simulink model "mpc_control_sim"  (R2019b)
settings: Solver=FixedStepAuto  StartTime=0.0  StopTime=72  FixedStep=h  RelTol=1e-3
values from neighbouring files (symbols this model uses):
  h = 0.1    [Example_9_Tracking_Delta_Input_Formulation.m]    (also in dyn_dist_mpc_control.m = 0.01; dyn_mpc_control.m = 0.01; dyn_pid_control.m = 0.01; init.m = 0.05)
  robot_sys_ss = lateral_2_dof_model_continuous_time(h, robot_vel, 0)    [Example_9_Tracking_Delta_Input_Formulation.m]    (also in dyn_dist_mpc_control.m = c2d(robot_sys_ss, h); dyn_mpc_control.m = c2d(robot_sys_ss, h); mpc_control.m = c2d(robot_sys_ss, h); pid_control.m = c2d(robot_sys_ss, h))
libraries: mpclib x1
settings Model: Creator=faaizz  LastModifiedBy=faaizz
settings SFSimCC: CustomCodeUndefinedFunction=UseInterfaceOnly

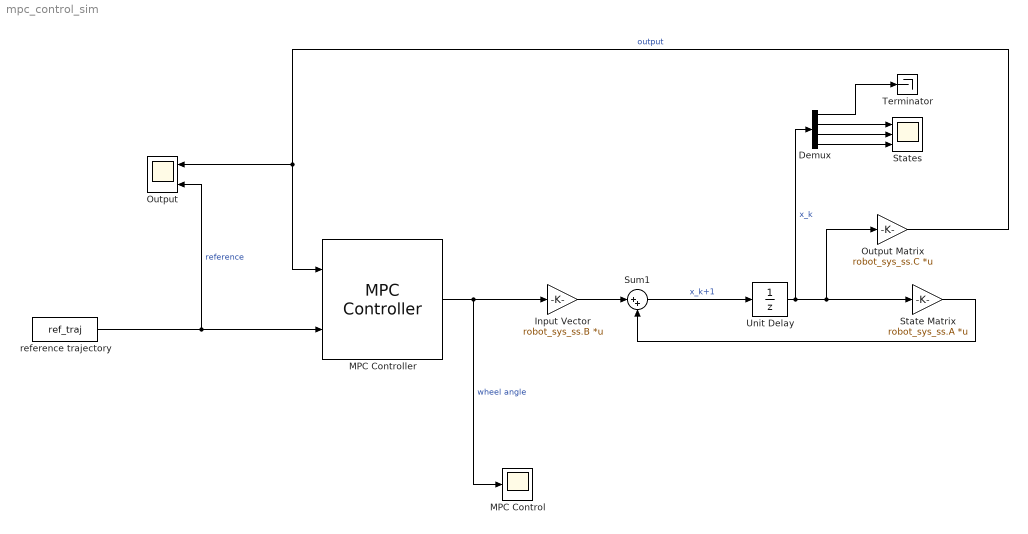
== system mpc_control_sim ==
  Demux : Demux
  Input Vector : Gain  Gain=robot_sys_ss.B  Multiplication=Matrix(K*u)
  MPC Control : Scope
  MPC Controller : mpclib/MPC Controller  SCDEnableBlockLinearizationSpecification=on  mpcobj=mpcobj  is_multiple=0  enable_value=0  return_u0=off  updateMPCinCallerWorkspace=on  md_inport=off  mv_inport=off  uref_inport=off  return_cost=off  return_mvseq=off  return_qpstatus=off  return_xseq=off  return_state=off  return_ovseq=off  state_inport=off  umin_inport=off  umax_inport=off  ymin_inport=off  ymax_inport=off  cc_inport=off  ywt_inport=off  uwt_inport=off  duwt_inport=off  rhoeps_inport=off  pm_inport=off  MaximumP=10  HorizonChoice=FixedHorizon  n_ts=0.1  n_p=100  n_mv=1  n_md=0  n_ud=0  n_mo=1  n_uo=0  BlockDataType=double  SampleTimeInherited=on  switch_inport=off
  Output : Scope  NumInputPorts=2
  Output Matrix : Gain  Gain=robot_sys_ss.C  Multiplication=Matrix(K*u)
  State Matrix : Gain  Gain=robot_sys_ss.A  Multiplication=Matrix(K*u)
  States : Scope  NumInputPorts=3
  Sum1 : Sum  Inputs=|++
  Terminator : Terminator
  Unit Delay : UnitDelay  SampleTime=-1  HasFrameUpgradeWarning=on
  reference trajectory : FromWorkspace  VariableName=ref_traj  SampleTime=h  OutputAfterFinalValue=Setting to zero
  wires:
  reference trajectory/1 -> Output/2, MPC Controller/2  "reference"
  MPC Controller/1 -> MPC Control/1, Input Vector/1  "wheel angle"
  Sum1/1 -> Unit Delay/1  "x_k+1"
  Unit Delay/1 -> Demux/1, State Matrix/1, Output Matrix/1  "x_k"
  Output Matrix/1 -> MPC Controller/1, Output/1  "output"
  State Matrix/1 -> Sum1/2
  Demux/2 -> States/1
  Demux/3 -> States/2
  Demux/4 -> States/3
  Input Vector/1 -> Sum1/1
  Demux/1 -> Terminator/1
